simulink model "Final_Simulation_with_Rough_Solver_Configuration"  (R2024b)
settings: Solver=VariableStepAuto  StartTime=0.0  StopTime=20  MaxStep=1e-4  RelTol=1e-3
libraries: spsDiodeLib x7, spsCurrentMeasurementLib x6, spsVoltageMeasurementLib x6, spsControlledVoltageSourceLib x3, simulink x3, spsSeriesRLCBranchLib x3, spsDCMachineLib x1, spsDCVoltageSourceLib x1, spsGroundLib x1, spsMosfetLib x1, spsPWMGeneratorDCDCLib x1, spsRMSLib x1
settings Model: Creator=sefer  LastModifiedBy=PC
settings DebuggingCC: IgnoredZcDiagnostic=none

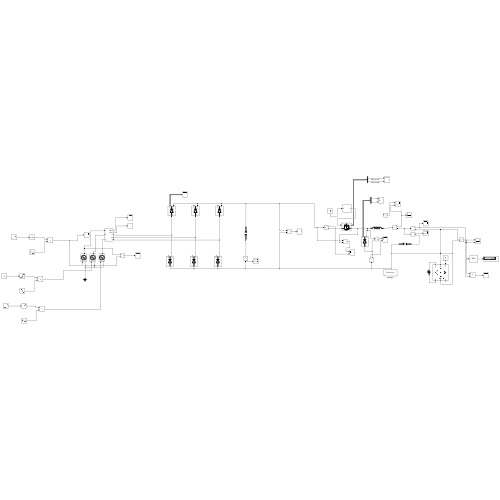
[thumbnail: Simulink's stored preview of the top-level diagram]
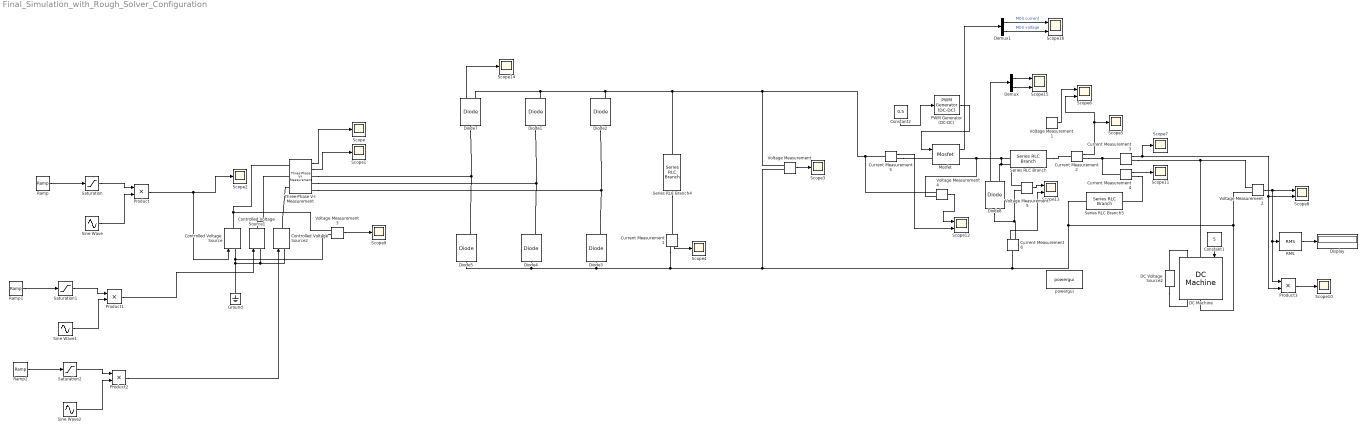
== system Final_Simulation_with_Rough_Solver_Configuration ==
  Constant1 : Constant  Value=5
  Constant2 : Constant  Value=0.5
  Controlled Voltage Source : spsControlledVoltageSourceLib/Controlled Voltage Source  Initialize=on  Source_Type=AC  Amplitude=0  Phase=0  Frequency=50  Measurements=None
  Controlled Voltage Source1 : spsControlledVoltageSourceLib/Controlled Voltage Source  Initialize=on  Source_Type=AC  Amplitude=0  Phase=0  Frequency=50  Measurements=None
  Controlled Voltage Source2 : spsControlledVoltageSourceLib/Controlled Voltage Source  Initialize=on  Source_Type=AC  Amplitude=0  Phase=0  Frequency=50  Measurements=None
  Current Measurement{1..6} (6 alike) : spsCurrentMeasurementLib/Current Measurement  PhasorSimulation=off  OutputType=Complex  PSBequivalent=0
  DC Machine : spsDCMachineLib/DC Machine  PresetModel=No  MechanicalLoad=Torque TL  FieldType=Wound  ShowDetailedParameters=on  MeasurementBus=off  RLa="[ 1.07  0.0245]"  RLf="[ 210  23]"  Laf=1.8  MachineConstant=Torque constant (N.m/A)  Ke=1.8  Kt=1.8  J=1  Bm=0  Tf=0  w0=1  Ifinit=1.04761904761905  TsPowergui=0  TsBlock=-1
  DC Voltage Source2 : spsDCVoltageSourceLib/DC Voltage Source  Amplitude=220  Measurements=None
  Demux : Demux  Outputs=2
  Demux1 : Demux  Outputs=2
  Diode{1..5,7} (6 alike) : spsDiodeLib/Diode  Ron=0.001  Lon=0  Vf=0  IC=0  UseSnubber=0  Rs=inf  Cs=0  Measurements=on
  Diode8 : spsDiodeLib/Diode  Ron=0  Lon=0  Vf=0  IC=0  UseSnubber=0  Rs=inf  Cs=0  Measurements=on
  Display : Display
  Ground : spsGroundLib/Ground  LConnTagsString=a
  Mosfet : spsMosfetLib/Mosfet  Ron=0.1  Lon=0  Rd=0.01  Vfd=0  IC=0  Rs=1e5  Cs=inf  Measurements=on
  PWM Generator (DC-DC) : spsPWMGeneratorDCDCLib/PWM Generator (DC-DC)  Fsw=5000  Ts=0
  Product{,1..3} (4 alike) : Product
  RMS : spsRMSLib/RMS  TrueRMS=on  Freq=60  RMSInit=120  Ts=0
  Ramp : simulink/Sources/Ramp  slope=0.2  start=0  InitialOutput=0
  Ramp1 : simulink/Sources/Ramp  slope=0.2  start=0  InitialOutput=0
  Ramp2 : simulink/Sources/Ramp  slope=0.2  start=0  InitialOutput=0
  Saturation : Saturate  UpperLimit=1
  Saturation1 : Saturate  UpperLimit=1
  Saturation2 : Saturate  UpperLimit=1
  Scope{,1..5,7,9..11,14} (11 alike) : Scope
  Scope{6,8,12..13,15..16} (6 alike) : Scope  NumInputPorts=2
  Series RLC Branch : spsSeriesRLCBranchLib/Series RLC Branch  LConnTagsString=__new0  RConnTagsString=__new0  BranchType=L  Resistance=1  Inductance=1e-3  SetiL0=off  InitialCurrent=0  Capacitance=1e-6  Setx0=off  InitialVoltage=0  Measurements=None
  Series RLC Branch4 : spsSeriesRLCBranchLib/Series RLC Branch  LConnTagsString=__new0  RConnTagsString=__new0  BranchType=C  Resistance=0.001  Inductance=1e-3  SetiL0=off  InitialCurrent=0  Capacitance=2000e-6  Setx0=off  InitialVoltage=0  Measurements=None
  Series RLC Branch5 : spsSeriesRLCBranchLib/Series RLC Branch  LConnTagsString=__new0  RConnTagsString=__new0  BranchType=C  Resistance=1  Inductance=1e-3  SetiL0=off  InitialCurrent=0  Capacitance=100e-6  Setx0=off  InitialVoltage=0  Measurements=None
  Sine Wave : Sin  Amplitude=105  Frequency=100*pi  SampleTime=0
  Sine Wave1 : Sin  Amplitude=105  Frequency=100*pi  Phase=2*pi/3  SampleTime=0
  Sine Wave2 : Sin  Amplitude=105  Frequency=100*pi  Phase=4*pi/3  SampleTime=0
  Three-Phase V-I Measurement : spsThreePhaseVIMeasurementLib/Three-Phase V-I Measurement  VoltageMeasurement=phase-to-ground  SetLabelV=off  LabelV=Vabc  Vpu=off  VpuLL=off  CurrentMeasurement=yes  SetLabelI=off  LabelI=Iabc  Ipu=off  Pbase=100e6  Vbase=500e3  OutputType=Complex  PhasorSimulation=off  PSBequivalent=0
  Voltage Measurement{,1..5} (6 alike) : spsVoltageMeasurementLib/Voltage Measurement  PhasorSimulation=off  OutputType=Complex  PSBequivalent=0
  powergui : sps_lib/powergui  Priority=1  SimulationMode=Continuous  SampleTime=1e-6  frequency=60  Iterations=50  frequencyindice=0  Pbase=100e6  ErrMax=1e-4  UnitsV=kV  UnitsW=MW  buscounter=0  FunctionMessages=off  echomessages=off  EnableUseOfTLC=off  CurrentSourceSwitches=off  DisableSnubberDevices=off  DisableRonSwitches=off  DisableVfSwitches=off  DisplayEquations=off  AutomaticDiscreteSolvers=off  SolverType=Tustin/Backward Euler (TBE)  Interpol=off  ExternalGateDelay=off  methode=off  Ts=100  x0status=blocks  SPID=on  SwTol=0  HookPort=off  NonlinearTolerance=1e-4  nMaxIteration=100  ContinueOnMaxIteration=off  RestoreLinks=warning  ResistiveCurrentMeasurement=off  Frange=[0:2:500]  Ylog=off  Xlog=on  ShowGrid=off  save=off  variable=ZData  structure=0  ZoomFFT=off  StartTime=0.0  cycles=1  DisplayStyle=1  fundamental=60  FreqAxis=off  MaxFrequency=1000  frequencyindicesteady=1  RmsSteady=1  display=off
  wires:
  Three-Phase V-I Measurement/1 -> Scope/1
  Three-Phase V-I Measurement/2 -> Scope1/1
  Voltage Measurement/1 -> Scope3/1
  Current Measurement1/1 -> Scope4/1
  Voltage Measurement2/1 -> Product3/1, RMS/1, Scope8/1
  Current Measurement3/1 -> Scope8/2, Product3/2, Scope7/1
  Current Measurement2/1 -> Scope6/2, Scope5/1
  Voltage Measurement1/1 -> Scope6/1
  Current Measurement4/1 -> Scope11/1
  Sine Wave/1 -> Product/2
  Ramp/1 -> Saturation/1
  Voltage Measurement3/1 -> Scope9/1
  Product/1 -> Controlled Voltage Source/1, Scope2/1
  Saturation/1 -> Product/1
  Saturation1/1 -> Product1/1
  Ramp1/1 -> Saturation1/1
  Sine Wave1/1 -> Product1/2
  Sine Wave2/1 -> Product2/2
  Ramp2/1 -> Saturation2/1
  Saturation2/1 -> Product2/1
  RMS/1 -> Display/1
  Constant1/1 -> DC Machine/1
  Product3/1 -> Scope10/1
  PWM Generator (DC-DC)/1 -> Mosfet/1
  Constant2/1 -> PWM Generator (DC-DC)/1
  Product1/1 -> Controlled Voltage Source1/1
  Product2/1 -> Controlled Voltage Source2/1
  Voltage Measurement4/1 -> Scope12/1
  Voltage Measurement5/1 -> Scope13/1
  Current Measurement5/1 -> Scope12/2
  Current Measurement6/1 -> Scope13/2
  Diode7/1 -> Scope14/1
  Diode8/1 -> Demux/1
  Demux/1 -> Scope15/1
  Demux/2 -> Scope15/2
  Demux1/1 -> Scope16/1  "MOS current"
  Demux1/2 -> Scope16/2  "MOS voltage"
  Mosfet/1 -> Demux1/1
  connections:
  Diode5/RConn1 -- Three-Phase V-I Measurement/RConn1 -- Diode7/LConn1
  Voltage Measurement2/LConn2 -- DC Machine/RConn1 -- Series RLC Branch5/RConn1 -- Current Measurement6/LConn1 -- Diode3/LConn1 -- Diode5/LConn1 -- Diode4/LConn1 -- Current Measurement1/RConn1 -- Voltage Measurement/LConn2
  Diode4/RConn1 -- Three-Phase V-I Measurement/RConn2 -- Diode1/LConn1
  Series RLC Branch4/RConn1 -- Current Measurement1/LConn1
  Diode1/RConn1 -- Diode7/RConn1 -- Diode2/RConn1 -- Voltage Measurement4/LConn1 -- Current Measurement5/LConn1 -- Voltage Measurement/LConn1 -- Series RLC Branch4/LConn1
  Diode3/RConn1 -- Three-Phase V-I Measurement/RConn3 -- Diode2/LConn1
  Current Measurement3/LConn1 -- Current Measurement4/LConn1 -- Current Measurement2/RConn1
  Current Measurement3/RConn1 -- DC Machine/LConn1 -- Voltage Measurement2/LConn1
  Diode8/RConn1 -- Voltage Measurement5/LConn1 -- Series RLC Branch/LConn1 -- Voltage Measurement4/LConn2 -- Mosfet/RConn1
  Current Measurement4/RConn1 -- Series RLC Branch5/LConn1
  Ground/LConn1 -- Voltage Measurement3/LConn2 -- Controlled Voltage Source/LConn1 -- Controlled Voltage Source2/LConn1 -- Controlled Voltage Source1/LConn1
  Controlled Voltage Source/RConn1 -- Voltage Measurement3/LConn1 -- Three-Phase V-I Measurement/LConn1
  Controlled Voltage Source1/RConn1 -- Three-Phase V-I Measurement/LConn2
  Controlled Voltage Source2/RConn1 -- Three-Phase V-I Measurement/LConn3
  DC Voltage Source2/RConn1 -- DC Machine/LConn2
  DC Voltage Source2/LConn1 -- DC Machine/RConn2
  Current Measurement5/RConn1 -- Mosfet/LConn1
  Voltage Measurement5/LConn2 -- Diode8/LConn1 -- Current Measurement6/RConn1
  Series RLC Branch/RConn1 -- Current Measurement2/LConn1
